simulink model "Slave_module_sim"  (R2017a)
settings: Solver=FixedStepDiscrete  StartTime=0.0  StopTime=10  FixedStep=1/fs  RelTol=1e-3
values from neighbouring files (symbols this model uses):
  FIR_Coef_m = fir1(N,fc/(0.5*fs),'low')    [Slave_module.m]
  fs = 100    [Slave_module.m]
undefined symbols (not defined in the file or in its folder): sigbuilder_block
settings Model: Creator=christian-dsa  LastModifiedBy=christian-dsa

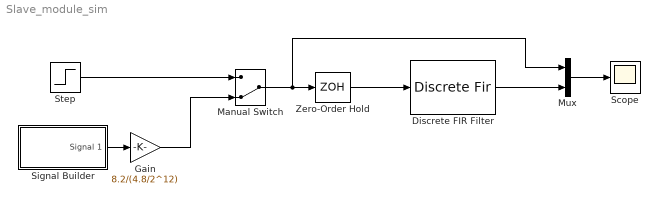
== system Slave_module_sim ==
  Discrete FIR Filter : DiscreteFir  Coefficients=FIR_Coef_m  InputProcessing=Columns as channels (frame based)  InitialStates=4  SampleTime=1/fs
  Gain : Gain  Gain=8.2/(4.8/2^12)
  Manual Switch : ManualSwitch  CurrentSetting=0
  Mux : Mux  Inputs=2
  Scope : Scope
  Signal Builder : Subsystem  Tag=STV Subsys  LoadFcn=sigbuilder_block('load');  StartFcn=sigbuilder_block('start');  StopFcn=sigbuilder_block('stop');  ClipboardFcn=sigbuilder_block('clipboard');  mask(Sigbuilder block){tuvar=[0:10]}
      mask help: Simulink:masks:SigbuilderBlock_MD
      mask init:
      | if ~strcmp(get_param(bdroot(gcbh),'SimulationStatus'),'stopped') tuvar = sigbuilder_block('maskInit'); end
      settings: CopyFcn=sigbuilder_block('copy');  DeleteFcn=sigbuilder_block('delete');  ModelCloseFcn=sigbuilder_block('modelClose');  PreSaveFcn=sigbuilder_block('preSave');  PauseFcn=sigbuilder_block('pause');  ContinueFcn=sigbuilder_block('continue');  NameChangeFcn=sigbuilder_block('namechange');  OpenFcn=sigbuilder_block('open',[431.25 193.5 562.5 393.75 ]);  CloseFcn=sigbuilder_block('close');
      mask Display: plot(0, 0, 100, 100,[2, 2, 32, 32, 2], [68, 8, 8, 68, 68],[32, 2], [38, 38], [32, 19, 2],[53, 60, 44], [32, 17, 17, 2],[16, 16, 31, 31]);txt = getActiveGroup(gcbh);text(2, 100, txt,'verticalAlignment', 'top');
  Step : Step  Before=4  After=4.01  SampleTime=0
  Zero-Order Hold : ZeroOrderHold  SampleTime=1/fs
  wires:
  Zero-Order Hold/1 -> Discrete FIR Filter/1
  Mux/1 -> Scope/1
  Discrete FIR Filter/1 -> Mux/2
  Manual Switch/1 -> Mux/1, Zero-Order Hold/1
  Step/1 -> Manual Switch/1
  Signal Builder/1(Signal 1) -> Gain/1
  Gain/1 -> Manual Switch/2

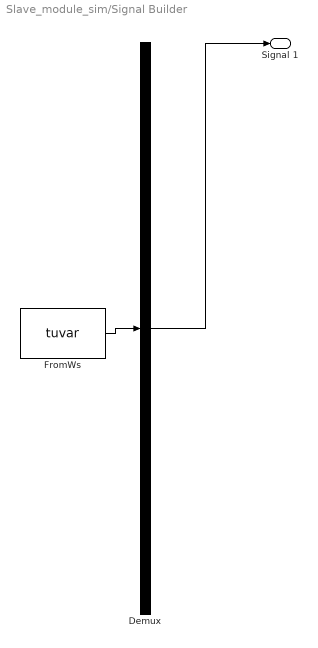
== system Slave_module_sim/Signal Builder ==
  Demux : Demux  Tag=STV Demux  Outputs=1
  FromWs : FromWorkspace  Tag=STV FromWs  VariableName=tuvar  SampleTime=0
      SigBuilderData=|
      | common.afterFinalStr = 'Extrapolate'
      | common.sampleTime = 0
      | dataSet.timeRange = [0 10]
      | dataSet.name = 'Group 1'
      | sbobj.Groups.Name = 'Group 1'
      | sbobj.Groups.Signals.Name = 'Signal 1'
      | sbobj.Groups.Signals.XData = [0 0.98 0.98 2 2.46 10]
      | sbobj.Groups.Signals.YData = [0.5 0.505 0.5122 0.5122 0.5 0.5]
  Signal 1 : Outport  Tag=STV Outport
  wires:
  Demux/1 -> Signal 1/1
  FromWs/1 -> Demux/1
